simulink model "holo"  (R2012b)
settings: Solver=FixedStepDiscrete  SolverMode=SingleTasking  StartTime=0.0  StopTime=160000  RelTol=1e-3
undefined symbols (not defined in the file): xlipgetpartsetting
libraries: xbsIndex_r4 x3470, casper_library_misc x43, simulink x18, dspsigops x12, casper_library_delays x8, xps_library x5, casper_library_multipliers x4
(part 13 of 36)

== system holo/dec_fir/fir_dbl_col7 ==
  real1 : Inport
  imag1 : Inport  Port=2
  real2 : Inport  Port=3
  imag2 : Inport  Port=4
  real3 : Inport  Port=5
  imag3 : Inport  Port=6
  real4 : Inport  Port=7
  imag4 : Inport  Port=8
  real_back1 : Inport  Port=9
  imag_back1 : Inport  Port=10
  real_back2 : Inport  Port=11
  imag_back2 : Inport  Port=12
  real_back3 : Inport  Port=13
  imag_back3 : Inport  Port=14
  real_back4 : Inport  Port=15
  imag_back4 : Inport  Port=16
  adder_tree1 : Subsystem  AncestorBlock=casper_library_misc/adder_tree  mask(adder_tree){n_inputs=4, latency=1, adder_imp=Behavioral, first_stage_hdl=on}
      mask prompts: n_inputs "Number of Inputs"; latency "Add Latency"; adder_imp "Adder implementation"; first_stage_hdl "Use behavioural HDL for first stage of adders"
      mask help:
      | Sums all inputs using a tree of adds and delays.
      |
      | Number of inputs: The number of inputs to the block to be summed
      | Add latency: The number of clock cycles to perform one addition (affects timing)..
      | Adder implementation: choice of fabric or DSP48E core, or behavioral HDL
      | Use behavioural HDL for first stage of adders: Causes the first stage of adders to be absorbed into DSP blocks if multipliers precede them (Virtex 5). Overrides Adder implementation
      mask init:
      | adder_tree_init(gcb, ...
      |     'n_inputs', n_inputs, ...
      |     'latency', latency, ...
      |     'adder_imp', adder_imp, ...
      |     'first_stage_hdl', first_stage_hdl);
      settings: AttributesFormatString=latency 2
      mask Help: eval('xlWeb(''http://casper.berkeley.edu/wiki/Adder_tree'')')
      mask TypeOptions adder_imp: Behavioral | Fabric | DSP48
  adder_tree2 : Subsystem  AncestorBlock=casper_library_misc/adder_tree  mask(adder_tree){n_inputs=4, latency=1, adder_imp=Behavioral, first_stage_hdl=on}
      mask prompts: n_inputs "Number of Inputs"; latency "Add Latency"; adder_imp "Adder implementation"; first_stage_hdl "Use behavioural HDL for first stage of adders"
      mask help:
      | Sums all inputs using a tree of adds and delays.
      |
      | Number of inputs: The number of inputs to the block to be summed
      | Add latency: The number of clock cycles to perform one addition (affects timing)..
      | Adder implementation: choice of fabric or DSP48E core, or behavioral HDL
      | Use behavioural HDL for first stage of adders: Causes the first stage of adders to be absorbed into DSP blocks if multipliers precede them (Virtex 5). Overrides Adder implementation
      mask init:
      | adder_tree_init(gcb, ...
      |     'n_inputs', n_inputs, ...
      |     'latency', latency, ...
      |     'adder_imp', adder_imp, ...
      |     'first_stage_hdl', first_stage_hdl);
      settings: AttributesFormatString=latency 2
      mask Help: eval('xlWeb(''http://casper.berkeley.edu/wiki/Adder_tree'')')
      mask TypeOptions adder_imp: Behavioral | Fabric | DSP48
  c1 : xbsIndex_r4/Constant  const=1  gui_display_data_type=Fixed-point  arith_type=Signed (2's comp)  n_bits=16  bin_pt=14  preci_type=Single  exp_width=8  frac_width=24  explicit_period=on  period=1  equ=P=C  opselect=C  inp2=PCIN>>17  opr=+  inp1=P  carry=CIN  dbl_ovrd=off  block_type=constant
  c2 : xbsIndex_r4/Constant  const=1  gui_display_data_type=Fixed-point  arith_type=Signed (2's comp)  n_bits=16  bin_pt=14  preci_type=Single  exp_width=8  frac_width=24  explicit_period=on  period=1  equ=P=C  opselect=C  inp2=PCIN>>17  opr=+  inp1=P  carry=CIN  dbl_ovrd=off  block_type=constant
  fir_dbl_tap1 : Subsystem  AncestorBlock=casper_library_downconverter/fir_dbl_tap  mask(fir_dbl_tap){factor=-0.0015248, add_latency=add_latency, mult_latency=mult_latency, coeff_bit_width=coeff_bit_width, coeff_bin_pt=coeff_bin_pt}
      mask prompts: add_latency "Add latency"; mult_latency "Mult latency"; coeff_bit_width "Coefficient bit width"; coeff_bin_pt "Coefficient binary point"
      mask init: same as holo/dec_fir/fir_dbl_col1/fir_dbl_tap1
      mask Help: eval('xlWeb(''http://casper.berkeley.edu/wiki/Fir_dbl_tap'')')
  fir_dbl_tap2 : Subsystem  AncestorBlock=casper_library_downconverter/fir_dbl_tap  mask(fir_dbl_tap){factor=-0.0009199, add_latency=add_latency, mult_latency=mult_latency, coeff_bit_width=coeff_bit_width, coeff_bin_pt=coeff_bin_pt}
      mask prompts: add_latency "Add latency"; mult_latency "Mult latency"; coeff_bit_width "Coefficient bit width"; coeff_bin_pt "Coefficient binary point"
      mask init: same as holo/dec_fir/fir_dbl_col1/fir_dbl_tap1
      mask Help: eval('xlWeb(''http://casper.berkeley.edu/wiki/Fir_dbl_tap'')')
  fir_dbl_tap3 : Subsystem  AncestorBlock=casper_library_downconverter/fir_dbl_tap  mask(fir_dbl_tap){factor=-0.00032795, add_latency=add_latency, mult_latency=mult_latency, coeff_bit_width=coeff_bit_width, coeff_bin_pt=coeff_bin_pt}
      mask prompts: add_latency "Add latency"; mult_latency "Mult latency"; coeff_bit_width "Coefficient bit width"; coeff_bin_pt "Coefficient binary point"
      mask init: same as holo/dec_fir/fir_dbl_col1/fir_dbl_tap1
      mask Help: eval('xlWeb(''http://casper.berkeley.edu/wiki/Fir_dbl_tap'')')
  fir_dbl_tap4 : Subsystem  AncestorBlock=casper_library_downconverter/fir_dbl_tap  mask(fir_dbl_tap){factor=0.00024561, add_latency=add_latency, mult_latency=mult_latency, coeff_bit_width=coeff_bit_width, coeff_bin_pt=coeff_bin_pt}
      mask prompts: add_latency "Add latency"; mult_latency "Mult latency"; coeff_bit_width "Coefficient bit width"; coeff_bin_pt "Coefficient binary point"
      mask init: same as holo/dec_fir/fir_dbl_col1/fir_dbl_tap1
      mask Help: eval('xlWeb(''http://casper.berkeley.edu/wiki/Fir_dbl_tap'')')
  term1 : Terminator
  term2 : Terminator
  real_out1 : Outport
  imag_out1 : Outport  Port=2
  real_out2 : Outport  Port=3
  imag_out2 : Outport  Port=4
  real_out3 : Outport  Port=5
  imag_out3 : Outport  Port=6
  real_out4 : Outport  Port=7
  imag_out4 : Outport  Port=8
  real_back_out1 : Outport  Port=9
  imag_back_out1 : Outport  Port=10
  real_back_out2 : Outport  Port=11
  imag_back_out2 : Outport  Port=12
  real_back_out3 : Outport  Port=13
  imag_back_out3 : Outport  Port=14
  real_back_out4 : Outport  Port=15
  imag_back_out4 : Outport  Port=16
  real_sum : Outport  Port=17
  imag_sum : Outport  Port=18
  wires:
  adder_tree1/1(sync_out) -> term1/1
  adder_tree2/1(sync_out) -> term2/1
  c1/1 -> adder_tree1/1(sync)
  c2/1 -> adder_tree2/1(sync)
  adder_tree1/2(dout) -> real_sum/1
  adder_tree2/2(dout) -> imag_sum/1
  real1/1 -> fir_dbl_tap1/1(a)
  imag1/1 -> fir_dbl_tap1/2(b)
  real_back4/1 -> fir_dbl_tap1/3(c)
  imag_back4/1 -> fir_dbl_tap1/4(d)
  fir_dbl_tap1/1(a_out) -> real_out1/1
  fir_dbl_tap1/2(b_out) -> imag_out1/1
  fir_dbl_tap1/3(c_out) -> real_back_out4/1
  fir_dbl_tap1/4(d_out) -> imag_back_out4/1
  fir_dbl_tap1/5(real) -> adder_tree1/2(din1)
  fir_dbl_tap1/6(imag) -> adder_tree2/2(din1)
  real2/1 -> fir_dbl_tap2/1(a)
  imag2/1 -> fir_dbl_tap2/2(b)
  real_back3/1 -> fir_dbl_tap2/3(c)
  imag_back3/1 -> fir_dbl_tap2/4(d)
  fir_dbl_tap2/1(a_out) -> real_out2/1
  fir_dbl_tap2/2(b_out) -> imag_out2/1
  fir_dbl_tap2/3(c_out) -> real_back_out3/1
  fir_dbl_tap2/4(d_out) -> imag_back_out3/1
  fir_dbl_tap2/5(real) -> adder_tree1/3(din2)
  fir_dbl_tap2/6(imag) -> adder_tree2/3(din2)
  real3/1 -> fir_dbl_tap3/1(a)
  imag3/1 -> fir_dbl_tap3/2(b)
  real_back2/1 -> fir_dbl_tap3/3(c)
  imag_back2/1 -> fir_dbl_tap3/4(d)
  fir_dbl_tap3/1(a_out) -> real_out3/1
  fir_dbl_tap3/2(b_out) -> imag_out3/1
  fir_dbl_tap3/3(c_out) -> real_back_out2/1
  fir_dbl_tap3/4(d_out) -> imag_back_out2/1
  fir_dbl_tap3/5(real) -> adder_tree1/4(din3)
  fir_dbl_tap3/6(imag) -> adder_tree2/4(din3)
  real4/1 -> fir_dbl_tap4/1(a)
  imag4/1 -> fir_dbl_tap4/2(b)
  real_back1/1 -> fir_dbl_tap4/3(c)
  imag_back1/1 -> fir_dbl_tap4/4(d)
  fir_dbl_tap4/1(a_out) -> real_out4/1
  fir_dbl_tap4/2(b_out) -> imag_out4/1
  fir_dbl_tap4/3(c_out) -> real_back_out1/1
  fir_dbl_tap4/4(d_out) -> imag_back_out1/1
  fir_dbl_tap4/5(real) -> adder_tree1/5(din4)
  fir_dbl_tap4/6(imag) -> adder_tree2/5(din4)

== system holo/dec_fir/fir_dbl_col8 ==
  real1 : Inport
  imag1 : Inport  Port=2
  real2 : Inport  Port=3
  imag2 : Inport  Port=4
  real3 : Inport  Port=5
  imag3 : Inport  Port=6
  real4 : Inport  Port=7
  imag4 : Inport  Port=8
  real_back1 : Inport  Port=9
  imag_back1 : Inport  Port=10
  real_back2 : Inport  Port=11
  imag_back2 : Inport  Port=12
  real_back3 : Inport  Port=13
  imag_back3 : Inport  Port=14
  real_back4 : Inport  Port=15
  imag_back4 : Inport  Port=16
  adder_tree1 : Subsystem  AncestorBlock=casper_library_misc/adder_tree  mask(adder_tree){n_inputs=4, latency=1, adder_imp=Behavioral, first_stage_hdl=on}
      mask prompts: n_inputs "Number of Inputs"; latency "Add Latency"; adder_imp "Adder implementation"; first_stage_hdl "Use behavioural HDL for first stage of adders"
      mask help:
      | Sums all inputs using a tree of adds and delays.
      |
      | Number of inputs: The number of inputs to the block to be summed
      | Add latency: The number of clock cycles to perform one addition (affects timing)..
      | Adder implementation: choice of fabric or DSP48E core, or behavioral HDL
      | Use behavioural HDL for first stage of adders: Causes the first stage of adders to be absorbed into DSP blocks if multipliers precede them (Virtex 5). Overrides Adder implementation
      mask init:
      | adder_tree_init(gcb, ...
      |     'n_inputs', n_inputs, ...
      |     'latency', latency, ...
      |     'adder_imp', adder_imp, ...
      |     'first_stage_hdl', first_stage_hdl);
      settings: AttributesFormatString=latency 2
      mask Help: eval('xlWeb(''http://casper.berkeley.edu/wiki/Adder_tree'')')
      mask TypeOptions adder_imp: Behavioral | Fabric | DSP48
  adder_tree2 : Subsystem  AncestorBlock=casper_library_misc/adder_tree  mask(adder_tree){n_inputs=4, latency=1, adder_imp=Behavioral, first_stage_hdl=on}
      mask prompts: n_inputs "Number of Inputs"; latency "Add Latency"; adder_imp "Adder implementation"; first_stage_hdl "Use behavioural HDL for first stage of adders"
      mask help:
      | Sums all inputs using a tree of adds and delays.
      |
      | Number of inputs: The number of inputs to the block to be summed
      | Add latency: The number of clock cycles to perform one addition (affects timing)..
      | Adder implementation: choice of fabric or DSP48E core, or behavioral HDL
      | Use behavioural HDL for first stage of adders: Causes the first stage of adders to be absorbed into DSP blocks if multipliers precede them (Virtex 5). Overrides Adder implementation
      mask init:
      | adder_tree_init(gcb, ...
      |     'n_inputs', n_inputs, ...
      |     'latency', latency, ...
      |     'adder_imp', adder_imp, ...
      |     'first_stage_hdl', first_stage_hdl);
      settings: AttributesFormatString=latency 2
      mask Help: eval('xlWeb(''http://casper.berkeley.edu/wiki/Adder_tree'')')
      mask TypeOptions adder_imp: Behavioral | Fabric | DSP48
  c1 : xbsIndex_r4/Constant  const=1  gui_display_data_type=Fixed-point  arith_type=Signed (2's comp)  n_bits=16  bin_pt=14  preci_type=Single  exp_width=8  frac_width=24  explicit_period=on  period=1  equ=P=C  opselect=C  inp2=PCIN>>17  opr=+  inp1=P  carry=CIN  dbl_ovrd=off  block_type=constant
  c2 : xbsIndex_r4/Constant  const=1  gui_display_data_type=Fixed-point  arith_type=Signed (2's comp)  n_bits=16  bin_pt=14  preci_type=Single  exp_width=8  frac_width=24  explicit_period=on  period=1  equ=P=C  opselect=C  inp2=PCIN>>17  opr=+  inp1=P  carry=CIN  dbl_ovrd=off  block_type=constant
  fir_dbl_tap1 : Subsystem  AncestorBlock=casper_library_downconverter/fir_dbl_tap  mask(fir_dbl_tap){factor=-0.0039413, add_latency=add_latency, mult_latency=mult_latency, coeff_bit_width=coeff_bit_width, coeff_bin_pt=coeff_bin_pt}
      mask prompts: add_latency "Add latency"; mult_latency "Mult latency"; coeff_bit_width "Coefficient bit width"; coeff_bin_pt "Coefficient binary point"
      mask init: same as holo/dec_fir/fir_dbl_col1/fir_dbl_tap1
      mask Help: eval('xlWeb(''http://casper.berkeley.edu/wiki/Fir_dbl_tap'')')
  fir_dbl_tap2 : Subsystem  AncestorBlock=casper_library_downconverter/fir_dbl_tap  mask(fir_dbl_tap){factor=-0.0033521, add_latency=add_latency, mult_latency=mult_latency, coeff_bit_width=coeff_bit_width, coeff_bin_pt=coeff_bin_pt}
      mask prompts: add_latency "Add latency"; mult_latency "Mult latency"; coeff_bit_width "Coefficient bit width"; coeff_bin_pt "Coefficient binary point"
      mask init: same as holo/dec_fir/fir_dbl_col1/fir_dbl_tap1
      mask Help: eval('xlWeb(''http://casper.berkeley.edu/wiki/Fir_dbl_tap'')')
  fir_dbl_tap3 : Subsystem  AncestorBlock=casper_library_downconverter/fir_dbl_tap  mask(fir_dbl_tap){factor=-0.0027479, add_latency=add_latency, mult_latency=mult_latency, coeff_bit_width=coeff_bit_width, coeff_bin_pt=coeff_bin_pt}
      mask prompts: add_latency "Add latency"; mult_latency "Mult latency"; coeff_bit_width "Coefficient bit width"; coeff_bin_pt "Coefficient binary point"
      mask init: same as holo/dec_fir/fir_dbl_col1/fir_dbl_tap1
      mask Help: eval('xlWeb(''http://casper.berkeley.edu/wiki/Fir_dbl_tap'')')
  fir_dbl_tap4 : Subsystem  AncestorBlock=casper_library_downconverter/fir_dbl_tap  mask(fir_dbl_tap){factor=-0.0021363, add_latency=add_latency, mult_latency=mult_latency, coeff_bit_width=coeff_bit_width, coeff_bin_pt=coeff_bin_pt}
      mask prompts: add_latency "Add latency"; mult_latency "Mult latency"; coeff_bit_width "Coefficient bit width"; coeff_bin_pt "Coefficient binary point"
      mask init: same as holo/dec_fir/fir_dbl_col1/fir_dbl_tap1
      mask Help: eval('xlWeb(''http://casper.berkeley.edu/wiki/Fir_dbl_tap'')')
  term1 : Terminator
  term2 : Terminator
  real_out1 : Outport
  imag_out1 : Outport  Port=2
  real_out2 : Outport  Port=3
  imag_out2 : Outport  Port=4
  real_out3 : Outport  Port=5
  imag_out3 : Outport  Port=6
  real_out4 : Outport  Port=7
  imag_out4 : Outport  Port=8
  real_back_out1 : Outport  Port=9
  imag_back_out1 : Outport  Port=10
  real_back_out2 : Outport  Port=11
  imag_back_out2 : Outport  Port=12
  real_back_out3 : Outport  Port=13
  imag_back_out3 : Outport  Port=14
  real_back_out4 : Outport  Port=15
  imag_back_out4 : Outport  Port=16
  real_sum : Outport  Port=17
  imag_sum : Outport  Port=18
  wires:
  adder_tree1/1(sync_out) -> term1/1
  adder_tree2/1(sync_out) -> term2/1
  c1/1 -> adder_tree1/1(sync)
  c2/1 -> adder_tree2/1(sync)
  adder_tree1/2(dout) -> real_sum/1
  adder_tree2/2(dout) -> imag_sum/1
  real1/1 -> fir_dbl_tap1/1(a)
  imag1/1 -> fir_dbl_tap1/2(b)
  real_back4/1 -> fir_dbl_tap1/3(c)
  imag_back4/1 -> fir_dbl_tap1/4(d)
  fir_dbl_tap1/1(a_out) -> real_out1/1
  fir_dbl_tap1/2(b_out) -> imag_out1/1
  fir_dbl_tap1/3(c_out) -> real_back_out4/1
  fir_dbl_tap1/4(d_out) -> imag_back_out4/1
  fir_dbl_tap1/5(real) -> adder_tree1/2(din1)
  fir_dbl_tap1/6(imag) -> adder_tree2/2(din1)
  real2/1 -> fir_dbl_tap2/1(a)
  imag2/1 -> fir_dbl_tap2/2(b)
  real_back3/1 -> fir_dbl_tap2/3(c)
  imag_back3/1 -> fir_dbl_tap2/4(d)
  fir_dbl_tap2/1(a_out) -> real_out2/1
  fir_dbl_tap2/2(b_out) -> imag_out2/1
  fir_dbl_tap2/3(c_out) -> real_back_out3/1
  fir_dbl_tap2/4(d_out) -> imag_back_out3/1
  fir_dbl_tap2/5(real) -> adder_tree1/3(din2)
  fir_dbl_tap2/6(imag) -> adder_tree2/3(din2)
  real3/1 -> fir_dbl_tap3/1(a)
  imag3/1 -> fir_dbl_tap3/2(b)
  real_back2/1 -> fir_dbl_tap3/3(c)
  imag_back2/1 -> fir_dbl_tap3/4(d)
  fir_dbl_tap3/1(a_out) -> real_out3/1
  fir_dbl_tap3/2(b_out) -> imag_out3/1
  fir_dbl_tap3/3(c_out) -> real_back_out2/1
  fir_dbl_tap3/4(d_out) -> imag_back_out2/1
  fir_dbl_tap3/5(real) -> adder_tree1/4(din3)
  fir_dbl_tap3/6(imag) -> adder_tree2/4(din3)
  real4/1 -> fir_dbl_tap4/1(a)
  imag4/1 -> fir_dbl_tap4/2(b)
  real_back1/1 -> fir_dbl_tap4/3(c)
  imag_back1/1 -> fir_dbl_tap4/4(d)
  fir_dbl_tap4/1(a_out) -> real_out4/1
  fir_dbl_tap4/2(b_out) -> imag_out4/1
  fir_dbl_tap4/3(c_out) -> real_back_out1/1
  fir_dbl_tap4/4(d_out) -> imag_back_out1/1
  fir_dbl_tap4/5(real) -> adder_tree1/5(din4)
  fir_dbl_tap4/6(imag) -> adder_tree2/5(din4)

== system holo/dec_fir/fir_dbl_col9 ==
  real1 : Inport
  imag1 : Inport  Port=2
  real2 : Inport  Port=3
  imag2 : Inport  Port=4
  real3 : Inport  Port=5
  imag3 : Inport  Port=6
  real4 : Inport  Port=7
  imag4 : Inport  Port=8
  real_back1 : Inport  Port=9
  imag_back1 : Inport  Port=10
  real_back2 : Inport  Port=11
  imag_back2 : Inport  Port=12
  real_back3 : Inport  Port=13
  imag_back3 : Inport  Port=14
  real_back4 : Inport  Port=15
  imag_back4 : Inport  Port=16
  adder_tree1 : Subsystem  AncestorBlock=casper_library_misc/adder_tree  mask(adder_tree){n_inputs=4, latency=1, adder_imp=Behavioral, first_stage_hdl=on}
      mask prompts: n_inputs "Number of Inputs"; latency "Add Latency"; adder_imp "Adder implementation"; first_stage_hdl "Use behavioural HDL for first stage of adders"
      mask help:
      | Sums all inputs using a tree of adds and delays.
      |
      | Number of inputs: The number of inputs to the block to be summed
      | Add latency: The number of clock cycles to perform one addition (affects timing)..
      | Adder implementation: choice of fabric or DSP48E core, or behavioral HDL
      | Use behavioural HDL for first stage of adders: Causes the first stage of adders to be absorbed into DSP blocks if multipliers precede them (Virtex 5). Overrides Adder implementation
      mask init:
      | adder_tree_init(gcb, ...
      |     'n_inputs', n_inputs, ...
      |     'latency', latency, ...
      |     'adder_imp', adder_imp, ...
      |     'first_stage_hdl', first_stage_hdl);
      settings: AttributesFormatString=latency 2
      mask Help: eval('xlWeb(''http://casper.berkeley.edu/wiki/Adder_tree'')')
      mask TypeOptions adder_imp: Behavioral | Fabric | DSP48
  adder_tree2 : Subsystem  AncestorBlock=casper_library_misc/adder_tree  mask(adder_tree){n_inputs=4, latency=1, adder_imp=Behavioral, first_stage_hdl=on}
      mask prompts: n_inputs "Number of Inputs"; latency "Add Latency"; adder_imp "Adder implementation"; first_stage_hdl "Use behavioural HDL for first stage of adders"
      mask help:
      | Sums all inputs using a tree of adds and delays.
      |
      | Number of inputs: The number of inputs to the block to be summed
      | Add latency: The number of clock cycles to perform one addition (affects timing)..
      | Adder implementation: choice of fabric or DSP48E core, or behavioral HDL
      | Use behavioural HDL for first stage of adders: Causes the first stage of adders to be absorbed into DSP blocks if multipliers precede them (Virtex 5). Overrides Adder implementation
      mask init:
      | adder_tree_init(gcb, ...
      |     'n_inputs', n_inputs, ...
      |     'latency', latency, ...
      |     'adder_imp', adder_imp, ...
      |     'first_stage_hdl', first_stage_hdl);
      settings: AttributesFormatString=latency 2
      mask Help: eval('xlWeb(''http://casper.berkeley.edu/wiki/Adder_tree'')')
      mask TypeOptions adder_imp: Behavioral | Fabric | DSP48
  c1 : xbsIndex_r4/Constant  const=1  gui_display_data_type=Fixed-point  arith_type=Signed (2's comp)  n_bits=16  bin_pt=14  preci_type=Single  exp_width=8  frac_width=24  explicit_period=on  period=1  equ=P=C  opselect=C  inp2=PCIN>>17  opr=+  inp1=P  carry=CIN  dbl_ovrd=off  block_type=constant
  c2 : xbsIndex_r4/Constant  const=1  gui_display_data_type=Fixed-point  arith_type=Signed (2's comp)  n_bits=16  bin_pt=14  preci_type=Single  exp_width=8  frac_width=24  explicit_period=on  period=1  equ=P=C  opselect=C  inp2=PCIN>>17  opr=+  inp1=P  carry=CIN  dbl_ovrd=off  block_type=constant
  fir_dbl_tap1 : Subsystem  AncestorBlock=casper_library_downconverter/fir_dbl_tap  mask(fir_dbl_tap){factor=-0.0059845, add_latency=add_latency, mult_latency=mult_latency, coeff_bit_width=coeff_bit_width, coeff_bin_pt=coeff_bin_pt}
      mask prompts: add_latency "Add latency"; mult_latency "Mult latency"; coeff_bit_width "Coefficient bit width"; coeff_bin_pt "Coefficient binary point"
      mask init: same as holo/dec_fir/fir_dbl_col1/fir_dbl_tap1
      mask Help: eval('xlWeb(''http://casper.berkeley.edu/wiki/Fir_dbl_tap'')')
  fir_dbl_tap2 : Subsystem  AncestorBlock=casper_library_downconverter/fir_dbl_tap  mask(fir_dbl_tap){factor=-0.0055375, add_latency=add_latency, mult_latency=mult_latency, coeff_bit_width=coeff_bit_width, coeff_bin_pt=coeff_bin_pt}
      mask prompts: add_latency "Add latency"; mult_latency "Mult latency"; coeff_bit_width "Coefficient bit width"; coeff_bin_pt "Coefficient binary point"
      mask init: same as holo/dec_fir/fir_dbl_col1/fir_dbl_tap1
      mask Help: eval('xlWeb(''http://casper.berkeley.edu/wiki/Fir_dbl_tap'')')
  fir_dbl_tap3 : Subsystem  AncestorBlock=casper_library_downconverter/fir_dbl_tap  mask(fir_dbl_tap){factor=-0.0050423, add_latency=add_latency, mult_latency=mult_latency, coeff_bit_width=coeff_bit_width, coeff_bin_pt=coeff_bin_pt}
      mask prompts: add_latency "Add latency"; mult_latency "Mult latency"; coeff_bit_width "Coefficient bit width"; coeff_bin_pt "Coefficient binary point"
      mask init: same as holo/dec_fir/fir_dbl_col1/fir_dbl_tap1
      mask Help: eval('xlWeb(''http://casper.berkeley.edu/wiki/Fir_dbl_tap'')')
  fir_dbl_tap4 : Subsystem  AncestorBlock=casper_library_downconverter/fir_dbl_tap  mask(fir_dbl_tap){factor=-0.0045074, add_latency=add_latency, mult_latency=mult_latency, coeff_bit_width=coeff_bit_width, coeff_bin_pt=coeff_bin_pt}
      mask prompts: add_latency "Add latency"; mult_latency "Mult latency"; coeff_bit_width "Coefficient bit width"; coeff_bin_pt "Coefficient binary point"
      mask init: same as holo/dec_fir/fir_dbl_col1/fir_dbl_tap1
      mask Help: eval('xlWeb(''http://casper.berkeley.edu/wiki/Fir_dbl_tap'')')
  term1 : Terminator
  term2 : Terminator
  real_out1 : Outport
  imag_out1 : Outport  Port=2
  real_out2 : Outport  Port=3
  imag_out2 : Outport  Port=4
  real_out3 : Outport  Port=5
  imag_out3 : Outport  Port=6
  real_out4 : Outport  Port=7
  imag_out4 : Outport  Port=8
  real_back_out1 : Outport  Port=9
  imag_back_out1 : Outport  Port=10
  real_back_out2 : Outport  Port=11
  imag_back_out2 : Outport  Port=12
  real_back_out3 : Outport  Port=13
  imag_back_out3 : Outport  Port=14
  real_back_out4 : Outport  Port=15
  imag_back_out4 : Outport  Port=16
  real_sum : Outport  Port=17
  imag_sum : Outport  Port=18
  wires:
  adder_tree1/1(sync_out) -> term1/1
  adder_tree2/1(sync_out) -> term2/1
  c1/1 -> adder_tree1/1(sync)
  c2/1 -> adder_tree2/1(sync)
  adder_tree1/2(dout) -> real_sum/1
  adder_tree2/2(dout) -> imag_sum/1
  real1/1 -> fir_dbl_tap1/1(a)
  imag1/1 -> fir_dbl_tap1/2(b)
  real_back4/1 -> fir_dbl_tap1/3(c)
  imag_back4/1 -> fir_dbl_tap1/4(d)
  fir_dbl_tap1/1(a_out) -> real_out1/1
  fir_dbl_tap1/2(b_out) -> imag_out1/1
  fir_dbl_tap1/3(c_out) -> real_back_out4/1
  fir_dbl_tap1/4(d_out) -> imag_back_out4/1
  fir_dbl_tap1/5(real) -> adder_tree1/2(din1)
  fir_dbl_tap1/6(imag) -> adder_tree2/2(din1)
  real2/1 -> fir_dbl_tap2/1(a)
  imag2/1 -> fir_dbl_tap2/2(b)
  real_back3/1 -> fir_dbl_tap2/3(c)
  imag_back3/1 -> fir_dbl_tap2/4(d)
  fir_dbl_tap2/1(a_out) -> real_out2/1
  fir_dbl_tap2/2(b_out) -> imag_out2/1
  fir_dbl_tap2/3(c_out) -> real_back_out3/1
  fir_dbl_tap2/4(d_out) -> imag_back_out3/1
  fir_dbl_tap2/5(real) -> adder_tree1/3(din2)
  fir_dbl_tap2/6(imag) -> adder_tree2/3(din2)
  real3/1 -> fir_dbl_tap3/1(a)
  imag3/1 -> fir_dbl_tap3/2(b)
  real_back2/1 -> fir_dbl_tap3/3(c)
  imag_back2/1 -> fir_dbl_tap3/4(d)
  fir_dbl_tap3/1(a_out) -> real_out3/1
  fir_dbl_tap3/2(b_out) -> imag_out3/1
  fir_dbl_tap3/3(c_out) -> real_back_out2/1
  fir_dbl_tap3/4(d_out) -> imag_back_out2/1
  fir_dbl_tap3/5(real) -> adder_tree1/4(din3)
  fir_dbl_tap3/6(imag) -> adder_tree2/4(din3)
  real4/1 -> fir_dbl_tap4/1(a)
  imag4/1 -> fir_dbl_tap4/2(b)
  real_back1/1 -> fir_dbl_tap4/3(c)
  imag_back1/1 -> fir_dbl_tap4/4(d)
  fir_dbl_tap4/1(a_out) -> real_out4/1
  fir_dbl_tap4/2(b_out) -> imag_out4/1
  fir_dbl_tap4/3(c_out) -> real_back_out1/1
  fir_dbl_tap4/4(d_out) -> imag_back_out1/1
  fir_dbl_tap4/5(real) -> adder_tree1/5(din4)
  fir_dbl_tap4/6(imag) -> adder_tree2/5(din4)

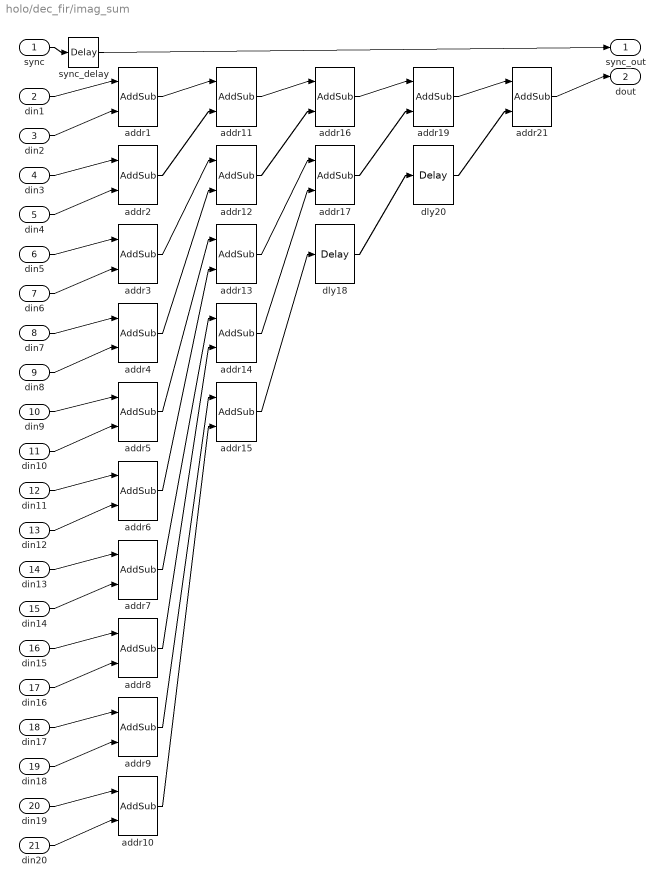
== system holo/dec_fir/imag_sum ==
  sync : Inport
  din1 : Inport  Port=2
  din2 : Inport  Port=3
  din3 : Inport  Port=4
  din4 : Inport  Port=5
  din5 : Inport  Port=6
  din6 : Inport  Port=7
  din7 : Inport  Port=8
  din8 : Inport  Port=9
  din9 : Inport  Port=10
  din10 : Inport  Port=11
  din11 : Inport  Port=12
  din12 : Inport  Port=13
  din13 : Inport  Port=14
  din14 : Inport  Port=15
  din15 : Inport  Port=16
  din16 : Inport  Port=17
  din17 : Inport  Port=18
  din18 : Inport  Port=19
  din19 : Inport  Port=20
  din20 : Inport  Port=21
  addr{1..10} (10 alike) : xbsIndex_r4/AddSub  mode=Addition  use_carryin=off  use_carryout=off  en=off  latency=1  precision=Full  arith_type=Unsigned  n_bits=16  bin_pt=14  quantization=Truncate  overflow=Wrap  dbl_ovrd=off  use_behavioral_HDL=off  hw_selection=Fabric  pipelined=on  use_rpm=on  block_type=addsub
  addr{11..17,19,21} (9 alike) : xbsIndex_r4/AddSub  mode=Addition  use_carryin=off  use_carryout=off  en=off  latency=1  precision=Full  arith_type=Unsigned  n_bits=16  bin_pt=14  quantization=Truncate  overflow=Wrap  dbl_ovrd=off  use_behavioral_HDL=on  hw_selection=Fabric  pipelined=on  use_rpm=on  block_type=addsub
  dly18 : xbsIndex_r4/Delay  rst=off  infoeditControl=Selection of Reset will increase slice count due to use of real FFs and instead of SRLs  en=off  latency=1  dbl_ovrd=off  reg_retiming=on  block_type=delay
  dly20 : xbsIndex_r4/Delay  rst=off  infoeditControl=Selection of Reset will increase slice count due to use of real FFs and instead of SRLs  en=off  latency=1  dbl_ovrd=off  reg_retiming=on  block_type=delay
  sync_delay : xbsIndex_r4/Delay  rst=off  infoeditControl=Selection of Reset will increase slice count due to use of real FFs and instead of SRLs  en=off  latency=5  dbl_ovrd=off  reg_retiming=on  block_type=delay
      settings: block_version=11.4
  sync_out : Outport
  dout : Outport  Port=2
  wires:
  sync/1 -> sync_delay/1
  sync_delay/1 -> sync_out/1
  din1/1 -> addr1/1
  din2/1 -> addr1/2
  din3/1 -> addr2/1
  din4/1 -> addr2/2
  din5/1 -> addr3/1
  din6/1 -> addr3/2
  din7/1 -> addr4/1
  din8/1 -> addr4/2
  din9/1 -> addr5/1
  din10/1 -> addr5/2
  din11/1 -> addr6/1
  din12/1 -> addr6/2
  din13/1 -> addr7/1
  din14/1 -> addr7/2
  din15/1 -> addr8/1
  din16/1 -> addr8/2
  din17/1 -> addr9/1
  din18/1 -> addr9/2
  din19/1 -> addr10/1
  din20/1 -> addr10/2
  addr1/1 -> addr11/1
  addr2/1 -> addr11/2
  addr3/1 -> addr12/1
  addr4/1 -> addr12/2
  addr5/1 -> addr13/1
  addr6/1 -> addr13/2
  addr7/1 -> addr14/1
  addr8/1 -> addr14/2
  addr9/1 -> addr15/1
  addr10/1 -> addr15/2
  addr11/1 -> addr16/1
  addr12/1 -> addr16/2
  addr13/1 -> addr17/1
  addr14/1 -> addr17/2
  addr15/1 -> dly18/1
  addr16/1 -> addr19/1
  addr17/1 -> addr19/2
  dly18/1 -> dly20/1
  addr19/1 -> addr21/1
  dly20/1 -> addr21/2
  addr21/1 -> dout/1

== system holo/dec_fir/real_sum ==
  sync : Inport
  din1 : Inport  Port=2
  din2 : Inport  Port=3
  din3 : Inport  Port=4
  din4 : Inport  Port=5
  din5 : Inport  Port=6
  din6 : Inport  Port=7
  din7 : Inport  Port=8
  din8 : Inport  Port=9
  din9 : Inport  Port=10
  din10 : Inport  Port=11
  din11 : Inport  Port=12
  din12 : Inport  Port=13
  din13 : Inport  Port=14
  din14 : Inport  Port=15
  din15 : Inport  Port=16
  din16 : Inport  Port=17
  din17 : Inport  Port=18
  din18 : Inport  Port=19
  din19 : Inport  Port=20
  din20 : Inport  Port=21
  addr{1..10} (10 alike) : xbsIndex_r4/AddSub  mode=Addition  use_carryin=off  use_carryout=off  en=off  latency=1  precision=Full  arith_type=Unsigned  n_bits=16  bin_pt=14  quantization=Truncate  overflow=Wrap  dbl_ovrd=off  use_behavioral_HDL=off  hw_selection=Fabric  pipelined=on  use_rpm=on  block_type=addsub
  addr{11..17,19,21} (9 alike) : xbsIndex_r4/AddSub  mode=Addition  use_carryin=off  use_carryout=off  en=off  latency=1  precision=Full  arith_type=Unsigned  n_bits=16  bin_pt=14  quantization=Truncate  overflow=Wrap  dbl_ovrd=off  use_behavioral_HDL=on  hw_selection=Fabric  pipelined=on  use_rpm=on  block_type=addsub
  dly18 : xbsIndex_r4/Delay  rst=off  infoeditControl=Selection of Reset will increase slice count due to use of real FFs and instead of SRLs  en=off  latency=1  dbl_ovrd=off  reg_retiming=on  block_type=delay
  dly20 : xbsIndex_r4/Delay  rst=off  infoeditControl=Selection of Reset will increase slice count due to use of real FFs and instead of SRLs  en=off  latency=1  dbl_ovrd=off  reg_retiming=on  block_type=delay
  sync_delay : xbsIndex_r4/Delay  rst=off  infoeditControl=Selection of Reset will increase slice count due to use of real FFs and instead of SRLs  en=off  latency=5  dbl_ovrd=off  reg_retiming=on  block_type=delay
      settings: block_version=11.4
  sync_out : Outport
  dout : Outport  Port=2
  wires:
  sync/1 -> sync_delay/1
  sync_delay/1 -> sync_out/1
  din1/1 -> addr1/1
  din2/1 -> addr1/2
  din3/1 -> addr2/1
  din4/1 -> addr2/2
  din5/1 -> addr3/1
  din6/1 -> addr3/2
  din7/1 -> addr4/1
  din8/1 -> addr4/2
  din9/1 -> addr5/1
  din10/1 -> addr5/2
  din11/1 -> addr6/1
  din12/1 -> addr6/2
  din13/1 -> addr7/1
  din14/1 -> addr7/2
  din15/1 -> addr8/1
  din16/1 -> addr8/2
  din17/1 -> addr9/1
  din18/1 -> addr9/2
  din19/1 -> addr10/1
  din20/1 -> addr10/2
  addr1/1 -> addr11/1
  addr2/1 -> addr11/2
  addr3/1 -> addr12/1
  addr4/1 -> addr12/2
  addr5/1 -> addr13/1
  addr6/1 -> addr13/2
  addr7/1 -> addr14/1
  addr8/1 -> addr14/2
  addr9/1 -> addr15/1
  addr10/1 -> addr15/2
  addr11/1 -> addr16/1
  addr12/1 -> addr16/2
  addr13/1 -> addr17/1
  addr14/1 -> addr17/2
  addr15/1 -> dly18/1
  addr16/1 -> addr19/1
  addr17/1 -> addr19/2
  dly18/1 -> dly20/1
  addr19/1 -> addr21/1
  dly20/1 -> addr21/2
  addr21/1 -> dout/1

== system holo/dec_fir1/fir_dbl_col1 ==
  real1 : Inport
  imag1 : Inport  Port=2
  real2 : Inport  Port=3
  imag2 : Inport  Port=4
  real3 : Inport  Port=5
  imag3 : Inport  Port=6
  real4 : Inport  Port=7
  imag4 : Inport  Port=8
  real_back1 : Inport  Port=9
  imag_back1 : Inport  Port=10
  real_back2 : Inport  Port=11
  imag_back2 : Inport  Port=12
  real_back3 : Inport  Port=13
  imag_back3 : Inport  Port=14
  real_back4 : Inport  Port=15
  imag_back4 : Inport  Port=16
  adder_tree1 : Subsystem  AncestorBlock=casper_library_misc/adder_tree  mask(adder_tree){n_inputs=4, latency=1, adder_imp=Behavioral, first_stage_hdl=on}
      mask prompts: n_inputs "Number of Inputs"; latency "Add Latency"; adder_imp "Adder implementation"; first_stage_hdl "Use behavioural HDL for first stage of adders"
      mask help:
      | Sums all inputs using a tree of adds and delays.
      |
      | Number of inputs: The number of inputs to the block to be summed
      | Add latency: The number of clock cycles to perform one addition (affects timing)..
      | Adder implementation: choice of fabric or DSP48E core, or behavioral HDL
      | Use behavioural HDL for first stage of adders: Causes the first stage of adders to be absorbed into DSP blocks if multipliers precede them (Virtex 5). Overrides Adder implementation
      mask init:
      | adder_tree_init(gcb, ...
      |     'n_inputs', n_inputs, ...
      |     'latency', latency, ...
      |     'adder_imp', adder_imp, ...
      |     'first_stage_hdl', first_stage_hdl);
      settings: AttributesFormatString=latency 2
      mask Help: eval('xlWeb(''http://casper.berkeley.edu/wiki/Adder_tree'')')
      mask TypeOptions adder_imp: Behavioral | Fabric | DSP48
  adder_tree2 : Subsystem  AncestorBlock=casper_library_misc/adder_tree  mask(adder_tree){n_inputs=4, latency=1, adder_imp=Behavioral, first_stage_hdl=on}
      mask prompts: n_inputs "Number of Inputs"; latency "Add Latency"; adder_imp "Adder implementation"; first_stage_hdl "Use behavioural HDL for first stage of adders"
      mask help:
      | Sums all inputs using a tree of adds and delays.
      |
      | Number of inputs: The number of inputs to the block to be summed
      | Add latency: The number of clock cycles to perform one addition (affects timing)..
      | Adder implementation: choice of fabric or DSP48E core, or behavioral HDL
      | Use behavioural HDL for first stage of adders: Causes the first stage of adders to be absorbed into DSP blocks if multipliers precede them (Virtex 5). Overrides Adder implementation
      mask init:
      | adder_tree_init(gcb, ...
      |     'n_inputs', n_inputs, ...
      |     'latency', latency, ...
      |     'adder_imp', adder_imp, ...
      |     'first_stage_hdl', first_stage_hdl);
      settings: AttributesFormatString=latency 2
      mask Help: eval('xlWeb(''http://casper.berkeley.edu/wiki/Adder_tree'')')
      mask TypeOptions adder_imp: Behavioral | Fabric | DSP48
  c1 : xbsIndex_r4/Constant  const=1  gui_display_data_type=Fixed-point  arith_type=Signed (2's comp)  n_bits=16  bin_pt=14  preci_type=Single  exp_width=8  frac_width=24  explicit_period=on  period=1  equ=P=C  opselect=C  inp2=PCIN>>17  opr=+  inp1=P  carry=CIN  dbl_ovrd=off  block_type=constant
  c2 : xbsIndex_r4/Constant  const=1  gui_display_data_type=Fixed-point  arith_type=Signed (2's comp)  n_bits=16  bin_pt=14  preci_type=Single  exp_width=8  frac_width=24  explicit_period=on  period=1  equ=P=C  opselect=C  inp2=PCIN>>17  opr=+  inp1=P  carry=CIN  dbl_ovrd=off  block_type=constant
  fir_dbl_tap1 : Subsystem  AncestorBlock=casper_library_downconverter/fir_dbl_tap  mask(fir_dbl_tap){factor=0.0082324, add_latency=add_latency, mult_latency=mult_latency, coeff_bit_width=coeff_bit_width, coeff_bin_pt=coeff_bin_pt}
      mask prompts: add_latency "Add latency"; mult_latency "Mult latency"; coeff_bit_width "Coefficient bit width"; coeff_bin_pt "Coefficient binary point"
      mask init: same as holo/dec_fir/fir_dbl_col1/fir_dbl_tap1
      mask Help: eval('xlWeb(''http://casper.berkeley.edu/wiki/Fir_dbl_tap'')')
  fir_dbl_tap2 : Subsystem  AncestorBlock=casper_library_downconverter/fir_dbl_tap  mask(fir_dbl_tap){factor=0.009013, add_latency=add_latency, mult_latency=mult_latency, coeff_bit_width=coeff_bit_width, coeff_bin_pt=coeff_bin_pt}
      mask prompts: add_latency "Add latency"; mult_latency "Mult latency"; coeff_bit_width "Coefficient bit width"; coeff_bin_pt "Coefficient binary point"
      mask init: same as holo/dec_fir/fir_dbl_col1/fir_dbl_tap1
      mask Help: eval('xlWeb(''http://casper.berkeley.edu/wiki/Fir_dbl_tap'')')
  fir_dbl_tap3 : Subsystem  AncestorBlock=casper_library_downconverter/fir_dbl_tap  mask(fir_dbl_tap){factor=0.0099508, add_latency=add_latency, mult_latency=mult_latency, coeff_bit_width=coeff_bit_width, coeff_bin_pt=coeff_bin_pt}
      mask prompts: add_latency "Add latency"; mult_latency "Mult latency"; coeff_bit_width "Coefficient bit width"; coeff_bin_pt "Coefficient binary point"
      mask init: same as holo/dec_fir/fir_dbl_col1/fir_dbl_tap1
      mask Help: eval('xlWeb(''http://casper.berkeley.edu/wiki/Fir_dbl_tap'')')
  fir_dbl_tap4 : Subsystem  AncestorBlock=casper_library_downconverter/fir_dbl_tap  mask(fir_dbl_tap){factor=-0.044769, add_latency=add_latency, mult_latency=mult_latency, coeff_bit_width=coeff_bit_width, coeff_bin_pt=coeff_bin_pt}
      mask prompts: add_latency "Add latency"; mult_latency "Mult latency"; coeff_bit_width "Coefficient bit width"; coeff_bin_pt "Coefficient binary point"
      mask init: same as holo/dec_fir/fir_dbl_col1/fir_dbl_tap1
      mask Help: eval('xlWeb(''http://casper.berkeley.edu/wiki/Fir_dbl_tap'')')
  term1 : Terminator
  term2 : Terminator
  real_out1 : Outport
  imag_out1 : Outport  Port=2
  real_out2 : Outport  Port=3
  imag_out2 : Outport  Port=4
  real_out3 : Outport  Port=5
  imag_out3 : Outport  Port=6
  real_out4 : Outport  Port=7
  imag_out4 : Outport  Port=8
  real_back_out1 : Outport  Port=9
  imag_back_out1 : Outport  Port=10
  real_back_out2 : Outport  Port=11
  imag_back_out2 : Outport  Port=12
  real_back_out3 : Outport  Port=13
  imag_back_out3 : Outport  Port=14
  real_back_out4 : Outport  Port=15
  imag_back_out4 : Outport  Port=16
  real_sum : Outport  Port=17
  imag_sum : Outport  Port=18
  wires:
  adder_tree1/1(sync_out) -> term1/1
  adder_tree2/1(sync_out) -> term2/1
  c1/1 -> adder_tree1/1(sync)
  c2/1 -> adder_tree2/1(sync)
  adder_tree1/2(dout) -> real_sum/1
  adder_tree2/2(dout) -> imag_sum/1
  real1/1 -> fir_dbl_tap1/1(a)
  imag1/1 -> fir_dbl_tap1/2(b)
  real_back4/1 -> fir_dbl_tap1/3(c)
  imag_back4/1 -> fir_dbl_tap1/4(d)
  fir_dbl_tap1/1(a_out) -> real_out1/1
  fir_dbl_tap1/2(b_out) -> imag_out1/1
  fir_dbl_tap1/3(c_out) -> real_back_out4/1
  fir_dbl_tap1/4(d_out) -> imag_back_out4/1
  fir_dbl_tap1/5(real) -> adder_tree1/2(din1)
  fir_dbl_tap1/6(imag) -> adder_tree2/2(din1)
  real2/1 -> fir_dbl_tap2/1(a)
  imag2/1 -> fir_dbl_tap2/2(b)
  real_back3/1 -> fir_dbl_tap2/3(c)
  imag_back3/1 -> fir_dbl_tap2/4(d)
  fir_dbl_tap2/1(a_out) -> real_out2/1
  fir_dbl_tap2/2(b_out) -> imag_out2/1
  fir_dbl_tap2/3(c_out) -> real_back_out3/1
  fir_dbl_tap2/4(d_out) -> imag_back_out3/1
  fir_dbl_tap2/5(real) -> adder_tree1/3(din2)
  fir_dbl_tap2/6(imag) -> adder_tree2/3(din2)
  real3/1 -> fir_dbl_tap3/1(a)
  imag3/1 -> fir_dbl_tap3/2(b)
  real_back2/1 -> fir_dbl_tap3/3(c)
  imag_back2/1 -> fir_dbl_tap3/4(d)
  fir_dbl_tap3/1(a_out) -> real_out3/1
  fir_dbl_tap3/2(b_out) -> imag_out3/1
  fir_dbl_tap3/3(c_out) -> real_back_out2/1
  fir_dbl_tap3/4(d_out) -> imag_back_out2/1
  fir_dbl_tap3/5(real) -> adder_tree1/4(din3)
  fir_dbl_tap3/6(imag) -> adder_tree2/4(din3)
  real4/1 -> fir_dbl_tap4/1(a)
  imag4/1 -> fir_dbl_tap4/2(b)
  real_back1/1 -> fir_dbl_tap4/3(c)
  imag_back1/1 -> fir_dbl_tap4/4(d)
  fir_dbl_tap4/1(a_out) -> real_out4/1
  fir_dbl_tap4/2(b_out) -> imag_out4/1
  fir_dbl_tap4/3(c_out) -> real_back_out1/1
  fir_dbl_tap4/4(d_out) -> imag_back_out1/1
  fir_dbl_tap4/5(real) -> adder_tree1/5(din4)
  fir_dbl_tap4/6(imag) -> adder_tree2/5(din4)

== system holo/dec_fir1/fir_dbl_col10 ==
  real1 : Inport
  imag1 : Inport  Port=2
  real2 : Inport  Port=3
  imag2 : Inport  Port=4
  real3 : Inport  Port=5
  imag3 : Inport  Port=6
  real4 : Inport  Port=7
  imag4 : Inport  Port=8
  real_back1 : Inport  Port=9
  imag_back1 : Inport  Port=10
  real_back2 : Inport  Port=11
  imag_back2 : Inport  Port=12
  real_back3 : Inport  Port=13
  imag_back3 : Inport  Port=14
  real_back4 : Inport  Port=15
  imag_back4 : Inport  Port=16
  adder_tree1 : Subsystem  AncestorBlock=casper_library_misc/adder_tree  mask(adder_tree){n_inputs=4, latency=1, adder_imp=Behavioral, first_stage_hdl=on}
      mask prompts: n_inputs "Number of Inputs"; latency "Add Latency"; adder_imp "Adder implementation"; first_stage_hdl "Use behavioural HDL for first stage of adders"
      mask help:
      | Sums all inputs using a tree of adds and delays.
      |
      | Number of inputs: The number of inputs to the block to be summed
      | Add latency: The number of clock cycles to perform one addition (affects timing)..
      | Adder implementation: choice of fabric or DSP48E core, or behavioral HDL
      | Use behavioural HDL for first stage of adders: Causes the first stage of adders to be absorbed into DSP blocks if multipliers precede them (Virtex 5). Overrides Adder implementation
      mask init:
      | adder_tree_init(gcb, ...
      |     'n_inputs', n_inputs, ...
      |     'latency', latency, ...
      |     'adder_imp', adder_imp, ...
      |     'first_stage_hdl', first_stage_hdl);
      settings: AttributesFormatString=latency 2
      mask Help: eval('xlWeb(''http://casper.berkeley.edu/wiki/Adder_tree'')')
      mask TypeOptions adder_imp: Behavioral | Fabric | DSP48
  adder_tree2 : Subsystem  AncestorBlock=casper_library_misc/adder_tree  mask(adder_tree){n_inputs=4, latency=1, adder_imp=Behavioral, first_stage_hdl=on}
      mask prompts: n_inputs "Number of Inputs"; latency "Add Latency"; adder_imp "Adder implementation"; first_stage_hdl "Use behavioural HDL for first stage of adders"
      mask help:
      | Sums all inputs using a tree of adds and delays.
      |
      | Number of inputs: The number of inputs to the block to be summed
      | Add latency: The number of clock cycles to perform one addition (affects timing)..
      | Adder implementation: choice of fabric or DSP48E core, or behavioral HDL
      | Use behavioural HDL for first stage of adders: Causes the first stage of adders to be absorbed into DSP blocks if multipliers precede them (Virtex 5). Overrides Adder implementation
      mask init:
      | adder_tree_init(gcb, ...
      |     'n_inputs', n_inputs, ...
      |     'latency', latency, ...
      |     'adder_imp', adder_imp, ...
      |     'first_stage_hdl', first_stage_hdl);
      settings: AttributesFormatString=latency 2
      mask Help: eval('xlWeb(''http://casper.berkeley.edu/wiki/Adder_tree'')')
      mask TypeOptions adder_imp: Behavioral | Fabric | DSP48
  c1 : xbsIndex_r4/Constant  const=1  gui_display_data_type=Fixed-point  arith_type=Signed (2's comp)  n_bits=16  bin_pt=14  preci_type=Single  exp_width=8  frac_width=24  explicit_period=on  period=1  equ=P=C  opselect=C  inp2=PCIN>>17  opr=+  inp1=P  carry=CIN  dbl_ovrd=off  block_type=constant
  c2 : xbsIndex_r4/Constant  const=1  gui_display_data_type=Fixed-point  arith_type=Signed (2's comp)  n_bits=16  bin_pt=14  preci_type=Single  exp_width=8  frac_width=24  explicit_period=on  period=1  equ=P=C  opselect=C  inp2=PCIN>>17  opr=+  inp1=P  carry=CIN  dbl_ovrd=off  block_type=constant
  fir_dbl_tap1 : Subsystem  AncestorBlock=casper_library_downconverter/fir_dbl_tap  mask(fir_dbl_tap){factor=-0.0071276, add_latency=add_latency, mult_latency=mult_latency, coeff_bit_width=coeff_bit_width, coeff_bin_pt=coeff_bin_pt}
      mask prompts: add_latency "Add latency"; mult_latency "Mult latency"; coeff_bit_width "Coefficient bit width"; coeff_bin_pt "Coefficient binary point"
      mask init: same as holo/dec_fir/fir_dbl_col1/fir_dbl_tap1
      mask Help: eval('xlWeb(''http://casper.berkeley.edu/wiki/Fir_dbl_tap'')')
  fir_dbl_tap2 : Subsystem  AncestorBlock=casper_library_downconverter/fir_dbl_tap  mask(fir_dbl_tap){factor=-0.0069543, add_latency=add_latency, mult_latency=mult_latency, coeff_bit_width=coeff_bit_width, coeff_bin_pt=coeff_bin_pt}
      mask prompts: add_latency "Add latency"; mult_latency "Mult latency"; coeff_bit_width "Coefficient bit width"; coeff_bin_pt "Coefficient binary point"
      mask init: same as holo/dec_fir/fir_dbl_col1/fir_dbl_tap1
      mask Help: eval('xlWeb(''http://casper.berkeley.edu/wiki/Fir_dbl_tap'')')
  fir_dbl_tap3 : Subsystem  AncestorBlock=casper_library_downconverter/fir_dbl_tap  mask(fir_dbl_tap){factor=-0.0067009, add_latency=add_latency, mult_latency=mult_latency, coeff_bit_width=coeff_bit_width, coeff_bin_pt=coeff_bin_pt}
      mask prompts: add_latency "Add latency"; mult_latency "Mult latency"; coeff_bit_width "Coefficient bit width"; coeff_bin_pt "Coefficient binary point"
      mask init: same as holo/dec_fir/fir_dbl_col1/fir_dbl_tap1
      mask Help: eval('xlWeb(''http://casper.berkeley.edu/wiki/Fir_dbl_tap'')')
  fir_dbl_tap4 : Subsystem  AncestorBlock=casper_library_downconverter/fir_dbl_tap  mask(fir_dbl_tap){factor=-0.006375, add_latency=add_latency, mult_latency=mult_latency, coeff_bit_width=coeff_bit_width, coeff_bin_pt=coeff_bin_pt}
      mask prompts: add_latency "Add latency"; mult_latency "Mult latency"; coeff_bit_width "Coefficient bit width"; coeff_bin_pt "Coefficient binary point"
      mask init: same as holo/dec_fir/fir_dbl_col1/fir_dbl_tap1
      mask Help: eval('xlWeb(''http://casper.berkeley.edu/wiki/Fir_dbl_tap'')')
  term1 : Terminator
  term2 : Terminator
  real_out1 : Outport
  imag_out1 : Outport  Port=2
  real_out2 : Outport  Port=3
  imag_out2 : Outport  Port=4
  real_out3 : Outport  Port=5
  imag_out3 : Outport  Port=6
  real_out4 : Outport  Port=7
  imag_out4 : Outport  Port=8
  real_back_out1 : Outport  Port=9
  imag_back_out1 : Outport  Port=10
  real_back_out2 : Outport  Port=11
  imag_back_out2 : Outport  Port=12
  real_back_out3 : Outport  Port=13
  imag_back_out3 : Outport  Port=14
  real_back_out4 : Outport  Port=15
  imag_back_out4 : Outport  Port=16
  real_sum : Outport  Port=17
  imag_sum : Outport  Port=18
  wires:
  adder_tree1/1(sync_out) -> term1/1
  adder_tree2/1(sync_out) -> term2/1
  c1/1 -> adder_tree1/1(sync)
  c2/1 -> adder_tree2/1(sync)
  adder_tree1/2(dout) -> real_sum/1
  adder_tree2/2(dout) -> imag_sum/1
  real1/1 -> fir_dbl_tap1/1(a)
  imag1/1 -> fir_dbl_tap1/2(b)
  real_back4/1 -> fir_dbl_tap1/3(c)
  imag_back4/1 -> fir_dbl_tap1/4(d)
  fir_dbl_tap1/1(a_out) -> real_out1/1
  fir_dbl_tap1/2(b_out) -> imag_out1/1
  fir_dbl_tap1/3(c_out) -> real_back_out4/1
  fir_dbl_tap1/4(d_out) -> imag_back_out4/1
  fir_dbl_tap1/5(real) -> adder_tree1/2(din1)
  fir_dbl_tap1/6(imag) -> adder_tree2/2(din1)
  real2/1 -> fir_dbl_tap2/1(a)
  imag2/1 -> fir_dbl_tap2/2(b)
  real_back3/1 -> fir_dbl_tap2/3(c)
  imag_back3/1 -> fir_dbl_tap2/4(d)
  fir_dbl_tap2/1(a_out) -> real_out2/1
  fir_dbl_tap2/2(b_out) -> imag_out2/1
  fir_dbl_tap2/3(c_out) -> real_back_out3/1
  fir_dbl_tap2/4(d_out) -> imag_back_out3/1
  fir_dbl_tap2/5(real) -> adder_tree1/3(din2)
  fir_dbl_tap2/6(imag) -> adder_tree2/3(din2)
  real3/1 -> fir_dbl_tap3/1(a)
  imag3/1 -> fir_dbl_tap3/2(b)
  real_back2/1 -> fir_dbl_tap3/3(c)
  imag_back2/1 -> fir_dbl_tap3/4(d)
  fir_dbl_tap3/1(a_out) -> real_out3/1
  fir_dbl_tap3/2(b_out) -> imag_out3/1
  fir_dbl_tap3/3(c_out) -> real_back_out2/1
  fir_dbl_tap3/4(d_out) -> imag_back_out2/1
  fir_dbl_tap3/5(real) -> adder_tree1/4(din3)
  fir_dbl_tap3/6(imag) -> adder_tree2/4(din3)
  real4/1 -> fir_dbl_tap4/1(a)
  imag4/1 -> fir_dbl_tap4/2(b)
  real_back1/1 -> fir_dbl_tap4/3(c)
  imag_back1/1 -> fir_dbl_tap4/4(d)
  fir_dbl_tap4/1(a_out) -> real_out4/1
  fir_dbl_tap4/2(b_out) -> imag_out4/1
  fir_dbl_tap4/3(c_out) -> real_back_out1/1
  fir_dbl_tap4/4(d_out) -> imag_back_out1/1
  fir_dbl_tap4/5(real) -> adder_tree1/5(din4)
  fir_dbl_tap4/6(imag) -> adder_tree2/5(din4)
